simulink model "q3"  (R2025a)
settings: Solver=VariableStepAuto  StartTime=0.0  StopTime=900  RelTol=1e-3
settings Model: Creator=dtemu  LastModifiedBy=dtemu

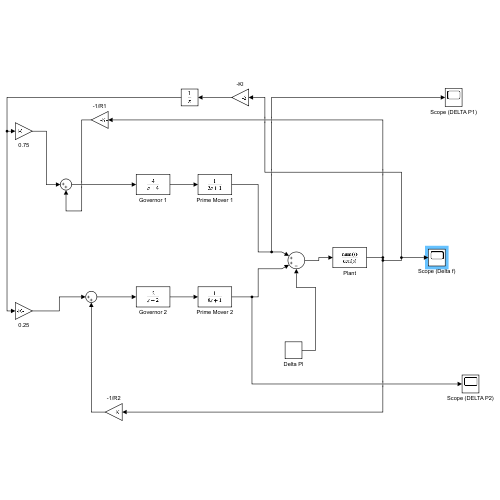
[thumbnail: Simulink's stored preview of the top-level diagram]
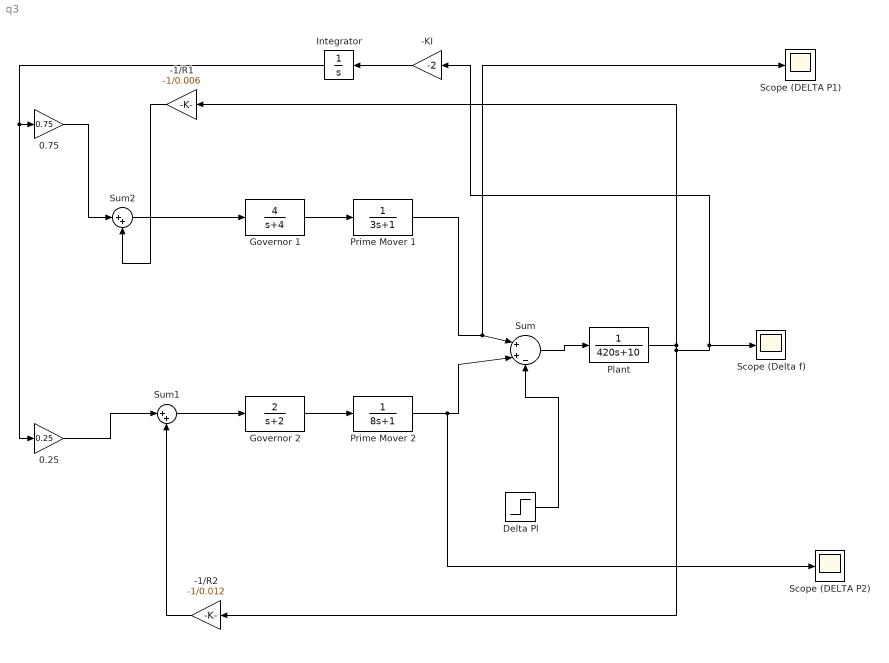
== system q3 ==
  -1/R1 : Gain  Gain=-1/0.006
  -1/R2 : Gain  Gain=-1/0.012
  -KI : Gain  Gain=-2
  0.25 : Gain  Gain=0.25
  0.75 : Gain  Gain=0.75
  Delta Pl : Step  Time=0  After=100  SampleTime=0
  Governor 1 : TransferFcn  Numerator=[4]  Denominator=[1 4]
  Governor 2 : TransferFcn  Numerator=[2]  Denominator=[1 2]
  Integrator : Integrator
  Plant : TransferFcn  Denominator=[420 10]
  Prime Mover 1 : TransferFcn  Denominator=[3 1]
  Prime Mover 2 : TransferFcn  Denominator=[8 1]
  Scope (DELTA P1) : Scope
      settings: ActiveDisplayYMinimum=-1  ActiveDisplayYMaximum=1  DataLoggingVariableName=ScopeData2
  Scope (DELTA P2) : Scope
      settings: ActiveDisplayYMinimum=-9.1343623216317518  ActiveDisplayYMaximum=39.336792897922535
  Scope (Delta f) : Scope
      settings: ActiveDisplayYMinimum=-0.80849893456627964  ActiveDisplayYMaximum=0.089833214951808835
  Sum : Sum  Inputs=|++-
  Sum1 : Sum  Inputs=|++
  Sum2 : Sum  Inputs=|++
  wires:
  -1/R1/1 -> Sum2/2
  Delta Pl/1 -> Sum/3
  -1/R2/1 -> Sum1/2
  Sum1/1 -> Governor 2/1
  -KI/1 -> Integrator/1
  0.75/1 -> Sum2/1
  Governor 2/1 -> Prime Mover 2/1
  Prime Mover 1/1 -> Scope (DELTA P1)/1, Sum/1
  Prime Mover 2/1 -> Scope (DELTA P2)/1, Sum/2
  Sum2/1 -> Governor 1/1
  Plant/1 -> -KI/1, Scope (Delta f)/1, -1/R2/1, -1/R1/1
  0.25/1 -> Sum1/1
  Sum/1 -> Plant/1
  Integrator/1 -> 0.25/1, 0.75/1
  Governor 1/1 -> Prime Mover 1/1
